simulink library "ddc_lo_lib"  (Simulink 6.2)
libraries: xbsIndex_r3 x4, ddc_lo_lib x1
settings Model: LastModifiedBy=aparsons

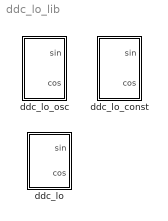
== system ddc_lo_lib ==
  ddc_lo : Subsystem  BlockChoice=ddc_lo_const
      settings: TemplateBlock=self  MemberBlocks=ddc_lo_const,ddc_lo_osc
  ddc_lo_const : Subsystem  mask(ddc_lo_const){BitWidth=18, Phase=0}
      mask prompts: BitWidth "Output Bitwidth"; Phase "Phase (0 to 2*pi)"
  ddc_lo_osc : Subsystem  mask(ddc_lo_osc){BitWidth=18, counter_step=1, counter_start=1, counter_width=4, latency=2}
      mask prompts: BitWidth "Output Bitwidth"; counter_step "counter step"; counter_start "counter start value"; counter_width "Counter Bitwidth"

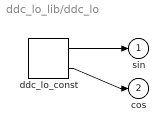
== system ddc_lo_lib/ddc_lo ==
  ddc_lo_const : ddc_lo_lib/ddc_lo_const  BitWidth=18  Phase=0
  sin : Outport
  cos : Outport  Port=2
  wires:
  ddc_lo_const/1 -> sin/1
  ddc_lo_const/2 -> cos/1

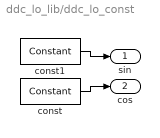
== system ddc_lo_lib/ddc_lo_const ==
  const : xbsIndex_r3/Constant  const=real(exp(Phase*1j))  equ=P=C  arith_type="Signed  (2's comp)"  n_bits=BitWidth  bin_pt=BitWidth - 1  opselect=C  inp2=PCIN>>17  opr=+  inp1=P  carry=CIN  iostate=0  explicit_period=on  period=1  dbl_ovrd=off
  const1 : xbsIndex_r3/Constant  const=-imag(exp(Phase*1j))  equ=P=C  arith_type="Signed  (2's comp)"  n_bits=BitWidth  bin_pt=BitWidth - 1  opselect=C  inp2=PCIN>>17  opr=+  inp1=P  carry=CIN  iostate=0  explicit_period=on  period=1  dbl_ovrd=off
  sin : Outport
  cos : Outport  Port=2
  wires:
  const1/1 -> sin/1
  const/1 -> cos/1

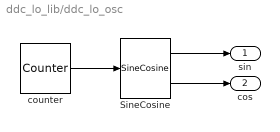
== system ddc_lo_lib/ddc_lo_osc ==
  SineCosine : xbsIndex_r3/SineCosine  mode=Sine and Cosine  neg_sin=on  neg_cos=off  n_bits=BitWidth  latency=latency  sym_output=off  explicit_period=off  period=1  en=off  dbl_ovrd=off  show_param=off  mem_type=Block RAM  pipeline=on  use_rpm=on  gen_core=off
      settings: xl_area=[0, 0, 0, 0, 0, 0, 0]
  counter : xbsIndex_r3/Counter  cnt_type=Free Running  n_bits=counter_width  bin_pt=0  arith_type=Unsigned  start_count=counter_start  cnt_to=Inf  cnt_by_val=counter_step  operation=Up  explicit_period=off  period=1  load_pin=off  rst=off  en=off  dbl_ovrd=off  show_param=off  use_rpm=on  gen_core=off
      settings: xl_area=[0, 0, 0, 0, 0, 0, 0]
  sin : Outport
  cos : Outport  Port=2
  wires:
  SineCosine/1 -> sin/1
  SineCosine/2 -> cos/1
  counter/1 -> SineCosine/1
